simulink model "spring_eq"  (R2020b)
settings: Solver=VariableStepAuto  StartTime=0.0  StopTime=50  MaxStep=0.01  RelTol=1e-3
values from neighbouring files (symbols this model uses):
  c = 2    [diff_equiations_code.m]    (also in spring_eq_code.m)
  f = 0.01    [electric_vehicle_edit.m]    (also in spring_eq_code.m = 2)
  k = 2    [diff_equiations_code.m]    (also in spring_eq_code.m = 100)
  m = 5    [diff_equiations_code.m]    (also in electric_vehicle_edit.m = 1500; spring_eq_code.m = 2)
libraries: dspsrcs4 x1
settings Model: Creator=amnessa  LastModifiedBy=amnessa

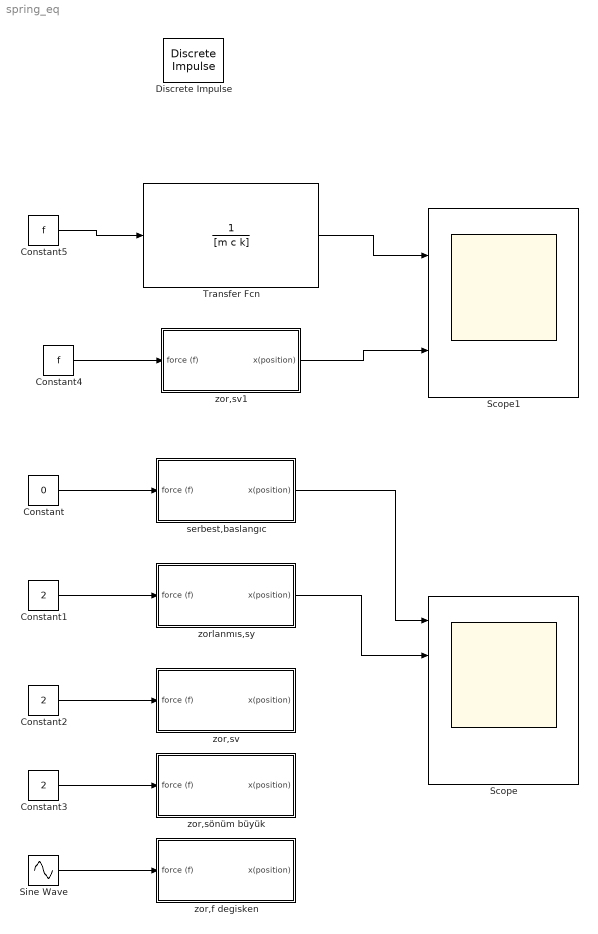
== system spring_eq ==
  Constant : Constant  Value=0
  Constant1 : Constant  Value=2
  Constant2 : Constant  Value=2
  Constant3 : Constant  Value=2
  Constant4 : Constant  Value=f
  Constant5 : Constant  Value=f
  Discrete Impulse : dspsrcs4/Discrete  Impulse  Delay=0  SampleTime=1  FrameSample=1  OutputFrames=off  dataType=double  isSigned=on  wordLen=16  udDataType=sfix(16)  fracBitsMode=Best precision  numFracBits=15  OutDataTypeStr=double  LastOutDataTypeStr=double
  Scope : Scope  NumInputPorts=5
  Scope1 : Scope  NumInputPorts=2
  Sine Wave : Sin  SampleTime=0
  Transfer Fcn : TransferFcn  Denominator=[m c k]
  serbest,baslangıc : Subsystem
  zor,f degisken : Subsystem
  zor,sv : Subsystem
  zor,sv1 : Subsystem
  zor,sönüm büyük : Subsystem
  zorlanmıs,sy : Subsystem
  wires:
  Constant/1 -> serbest,baslangıc/1(force (f))
  Constant1/1 -> zorlanmıs,sy/1(force (f))
  Constant2/1 -> zor,sv/1(force (f))
  Constant3/1 -> zor,sönüm büyük/1(force (f))
  Sine Wave/1 -> zor,f degisken/1(force (f))
  zorlanmıs,sy/1(x(position)) -> Scope/2
  serbest,baslangıc/1(x(position)) -> Scope/1
  Constant4/1 -> zor,sv1/1(force (f))
  Constant5/1 -> Transfer Fcn/1
  Transfer Fcn/1 -> Scope1/1
  zor,sv1/1(x(position)) -> Scope1/2

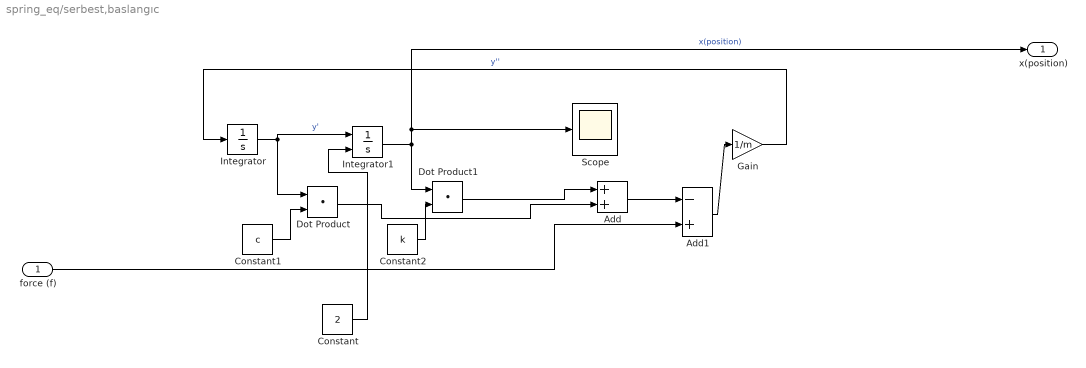
== system spring_eq/serbest,baslangıc ==
  force (f) : Inport
  Add : Sum
  Add1 : Sum  Inputs=-+
  Constant : Constant  Value=2
  Constant1 : Constant  Value=c
  Constant2 : Constant  Value=k
  Dot Product : DotProduct  InputSameDT=on  OutDataTypeStr=Inherit: Inherit via internal rule
  Dot Product1 : DotProduct  InputSameDT=on  OutDataTypeStr=Inherit: Inherit via internal rule
  Gain : Gain  Gain=1/m
  Integrator : Integrator
  Integrator1 : Integrator  InitialConditionSource=external
  Scope : Scope
  x(position) : Outport
  wires:
  Integrator/1 -> Dot Product/1, Integrator1/1  "y'"
  Add/1 -> Add1/1
  Gain/1 -> Integrator/1  "y''"
  Constant2/1 -> Dot Product1/2
  Integrator1/1 -> x(position)/1, Scope/1, Dot Product1/1  "x(position)"
  Constant1/1 -> Dot Product/2
  Dot Product/1 -> Add/2
  Add1/1 -> Gain/1
  Dot Product1/1 -> Add/1
  force (f)/1 -> Add1/2
  Constant/1 -> Integrator1/2

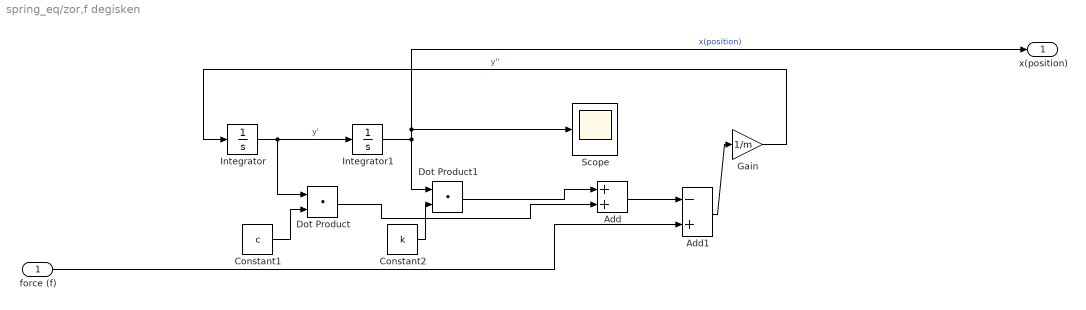
== system spring_eq/zor,f degisken ==
  force (f) : Inport
  Add : Sum
  Add1 : Sum  Inputs=-+
  Constant1 : Constant  Value=c
  Constant2 : Constant  Value=k
  Dot Product : DotProduct  InputSameDT=on  OutDataTypeStr=Inherit: Inherit via internal rule
  Dot Product1 : DotProduct  InputSameDT=on  OutDataTypeStr=Inherit: Inherit via internal rule
  Gain : Gain  Gain=1/m
  Integrator : Integrator
  Integrator1 : Integrator
  Scope : Scope
  x(position) : Outport
  wires:
  Integrator/1 -> Dot Product/1, Integrator1/1  "y'"
  Add/1 -> Add1/1
  Gain/1 -> Integrator/1  "y''"
  Constant2/1 -> Dot Product1/2
  Integrator1/1 -> x(position)/1, Scope/1, Dot Product1/1  "x(position)"
  Constant1/1 -> Dot Product/2
  Dot Product/1 -> Add/2
  Add1/1 -> Gain/1
  Dot Product1/1 -> Add/1
  force (f)/1 -> Add1/2

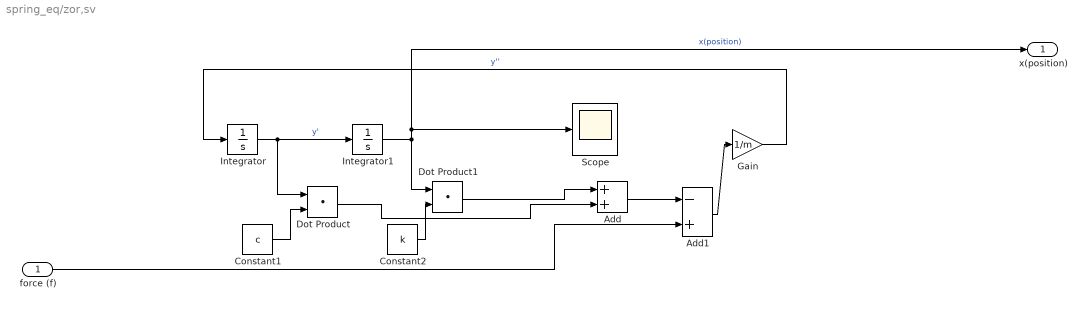
== system spring_eq/zor,sv ==
  force (f) : Inport
  Add : Sum
  Add1 : Sum  Inputs=-+
  Constant1 : Constant  Value=c
  Constant2 : Constant  Value=k
  Dot Product : DotProduct  InputSameDT=on  OutDataTypeStr=Inherit: Inherit via internal rule
  Dot Product1 : DotProduct  InputSameDT=on  OutDataTypeStr=Inherit: Inherit via internal rule
  Gain : Gain  Gain=1/m
  Integrator : Integrator
  Integrator1 : Integrator
  Scope : Scope
  x(position) : Outport
  wires:
  Integrator/1 -> Dot Product/1, Integrator1/1  "y'"
  Add/1 -> Add1/1
  Gain/1 -> Integrator/1  "y''"
  Constant2/1 -> Dot Product1/2
  Integrator1/1 -> x(position)/1, Scope/1, Dot Product1/1  "x(position)"
  Constant1/1 -> Dot Product/2
  Dot Product/1 -> Add/2
  Add1/1 -> Gain/1
  Dot Product1/1 -> Add/1
  force (f)/1 -> Add1/2

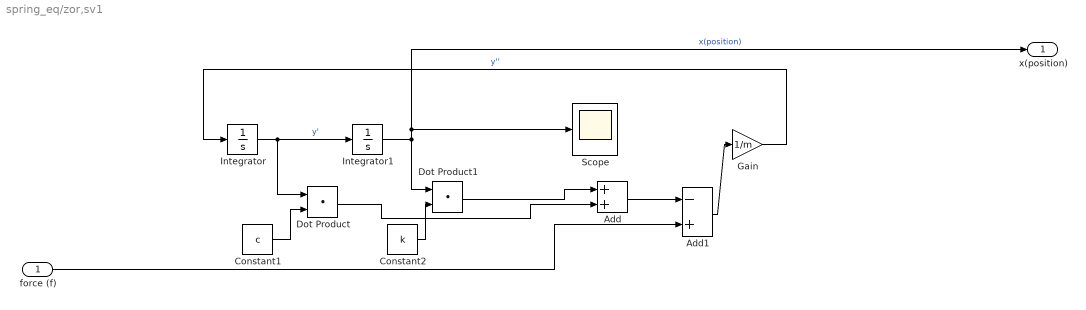
== system spring_eq/zor,sv1 ==
  force (f) : Inport
  Add : Sum
  Add1 : Sum  Inputs=-+
  Constant1 : Constant  Value=c
  Constant2 : Constant  Value=k
  Dot Product : DotProduct  InputSameDT=on  OutDataTypeStr=Inherit: Inherit via internal rule
  Dot Product1 : DotProduct  InputSameDT=on  OutDataTypeStr=Inherit: Inherit via internal rule
  Gain : Gain  Gain=1/m
  Integrator : Integrator
  Integrator1 : Integrator
  Scope : Scope
  x(position) : Outport
  wires:
  force (f)/1 -> Add1/2
  Dot Product1/1 -> Add/1
  Add1/1 -> Gain/1
  Dot Product/1 -> Add/2
  Constant1/1 -> Dot Product/2
  Integrator1/1 -> Dot Product1/1, Scope/1, x(position)/1  "x(position)"
  Constant2/1 -> Dot Product1/2
  Gain/1 -> Integrator/1  "y''"
  Add/1 -> Add1/1
  Integrator/1 -> Integrator1/1, Dot Product/1  "y'"

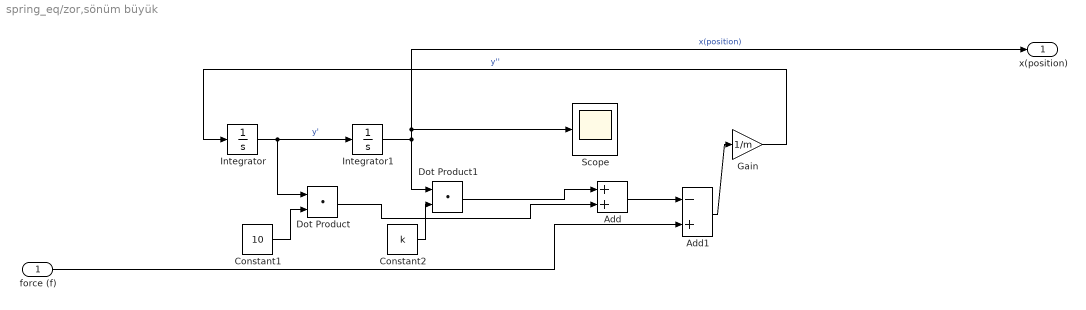
== system spring_eq/zor,sönüm büyük ==
  force (f) : Inport
  Add : Sum
  Add1 : Sum  Inputs=-+
  Constant1 : Constant  Value=10
  Constant2 : Constant  Value=k
  Dot Product : DotProduct  InputSameDT=on  OutDataTypeStr=Inherit: Inherit via internal rule
  Dot Product1 : DotProduct  InputSameDT=on  OutDataTypeStr=Inherit: Inherit via internal rule
  Gain : Gain  Gain=1/m
  Integrator : Integrator
  Integrator1 : Integrator
  Scope : Scope
  x(position) : Outport
  wires:
  force (f)/1 -> Add1/2
  Dot Product1/1 -> Add/1
  Add1/1 -> Gain/1
  Dot Product/1 -> Add/2
  Constant1/1 -> Dot Product/2
  Integrator1/1 -> Dot Product1/1, Scope/1, x(position)/1  "x(position)"
  Constant2/1 -> Dot Product1/2
  Gain/1 -> Integrator/1  "y''"
  Add/1 -> Add1/1
  Integrator/1 -> Integrator1/1, Dot Product/1  "y'"

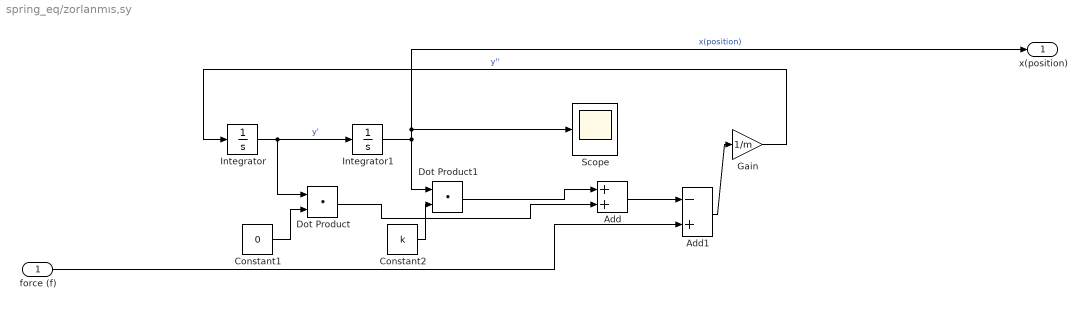
== system spring_eq/zorlanmıs,sy ==
  force (f) : Inport
  Add : Sum
  Add1 : Sum  Inputs=-+
  Constant1 : Constant  Value=0
  Constant2 : Constant  Value=k
  Dot Product : DotProduct  InputSameDT=on  OutDataTypeStr=Inherit: Inherit via internal rule
  Dot Product1 : DotProduct  InputSameDT=on  OutDataTypeStr=Inherit: Inherit via internal rule
  Gain : Gain  Gain=1/m
  Integrator : Integrator
  Integrator1 : Integrator
  Scope : Scope
  x(position) : Outport
  wires:
  force (f)/1 -> Add1/2
  Dot Product1/1 -> Add/1
  Add1/1 -> Gain/1
  Dot Product/1 -> Add/2
  Constant1/1 -> Dot Product/2
  Integrator1/1 -> Dot Product1/1, Scope/1, x(position)/1  "x(position)"
  Constant2/1 -> Dot Product1/2
  Gain/1 -> Integrator/1  "y''"
  Add/1 -> Add1/1
  Integrator/1 -> Integrator1/1, Dot Product/1  "y'"
